simulink model "eHStest"  (R2020b)
settings: Solver=ode4  StartTime=0.0  StopTime=inf  FixedStep=Ts  RelTol=1e-3
PostLoadFcn:
  | Two_Level_Inverter_params;
InitFcn:
  | Two_Level_Inverter_params;
values from neighbouring files (symbols this model uses):
  FilterDenominator = discreteFilterc.Denominator{1}    [Two_Level_Inverter_params.m]
  FilterNumerator = discreteFilterc.Numerator{1}(2)    [Two_Level_Inverter_params.m]
  Ts = 50e-6 * 5*4    (= 0.001)    [Two_Level_Inverter_params.m]
  Udc = 650    [Two_Level_Inverter_params.m]
undefined symbols (not defined in the file or in its folder): eHSx128m_Gen4_C0D8FBCEC0D8FBCE, EX, VC707_2
libraries: powerlib_meascontrol x16, dspstat3 x8, rtlab x6, rteventslib x6, rtio_opalrt_common x5, efs_cpuhilios_crtl_lib x2, cpuhilios_lib x1, ehsCpuLib x1
settings Model: Creator=Jun Zhang  LastModifiedBy=Jun.Zhang
settings SolverCC: SolverJacobianMethodControl=FullAnalytical
settings OptimizationCC: BlockReduction=off  OptimizeBlockIOStorage=off  LocalBlockOutputs=off

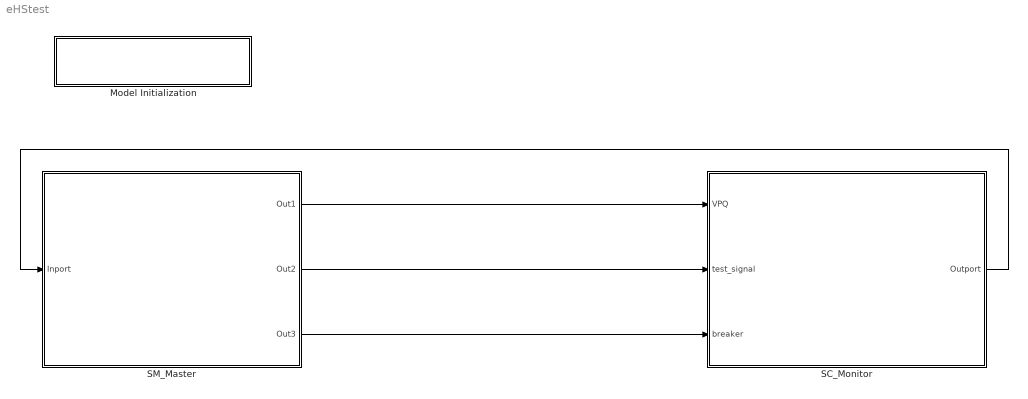
== system eHStest ==
  Model Initialization : Subsystem  AncestorBlock=artemis/Tools /Misc/Model Initialization  mask(Model Functions){InitFcnX=Two_Level_Inverter_params;, prel=off, posl=on, inif=on, strf=off}
      mask prompts: InitFcnX "Initialisation"; prel "Preload Function"; posl "PostLoad Function"; inif "InitFcn"; strf "StartFcn"
      mask init:
      | currentBlock = gcb;
      | root = bdroot(currentBlock);
      | 
      | if ~strcmp(get_param(root,'BlockDiagramType'),'library')
      |     if prel==1
      |         set_param(root, 'PreLoadFcn', InitFcnX);
      |     else
      |         set_param(root, 'PreLoadFcn', '');
      |     end
      |     if inif==1
      |         set_param(root, 'InitFcn', InitFcnX);
      |     else
      |         set_param(root, 'InitFcn', '');
      |     end
      |     if strf==1
      |         set_param(root, 'StartFcn', InitFcnX);
      |     else
      |         set_param(root, 'StartFcn', '');
      |     end
      |     if posl==1
      |         set_param(root, 'PostLoadFcn', InitFcnX);
      |     else
      |         set_param(root, 'PostLoadFcn', '');
      |     end
      | end
      | 
      | pos = get_param(currentBlock, 'Position');
      | width = pos(3) - pos(1); height = pos(4) - pos(2);
      | txt = [ upper(root) '\n' '- InitFcn. . . . . '  get_param(root, 'InitFcn') ];
      settings: CopyFcn=set_param(gcb,'LinkStatus','inactive')
      mask Display: text(5, height*0.5, txt, 'horizontalAlignment', 'left', 'verticalAlignment', 'middle') ;
  SC_Monitor : Subsystem
  SM_Master : Subsystem
  wires:
  SM_Master/1(Out1) -> SC_Monitor/1(VPQ)
  SM_Master/3(Out3) -> SC_Monitor/3(breaker)
  SM_Master/2(Out2) -> SC_Monitor/2(test_signal)
  SC_Monitor/1(Outport) -> SM_Master/1(Inport)

== system eHStest/Model Initialization ==

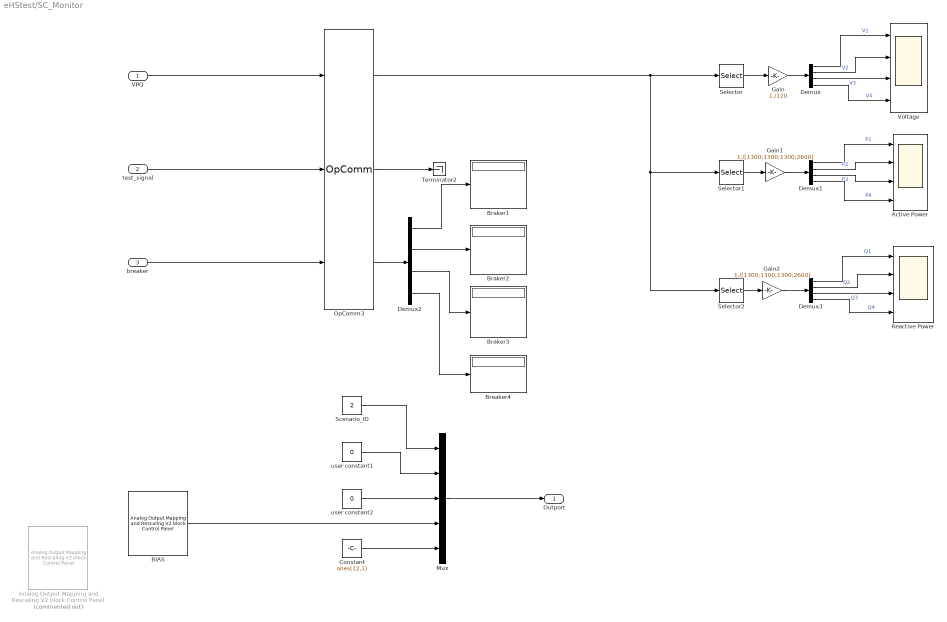
== system eHStest/SC_Monitor ==
  VPQ : Inport
  test_signal : Inport  Port=2
  breaker : Inport  Port=3
  Active Power : Scope  NumInputPorts=4
  Analog Output Mapping and Rescaling V2 block Control Panel : efs_cpuhilios_crtl_lib/Analog Output Mapping and  Rescaling V2 block Control Panel  Commented=on  controllerName='OpCtrl'  aomrVersion=V2  numberOfSourcesV1=0  numberOfSourcesV2=1  inputName0=Custom List  list0={'UserAnalogOut1', 'UserAnalogOut2', 'UserAnalogOut3', 'UserAnalogOut4'}  inputName1=Custom List  list1={'ehs1.Y1', 'ehs1.Y2', 'ehs1.Y3', 'ehs1.Y4', 'ehs1.Y5', 'ehs1.Y6', 'ehs1.Y7', 'ehs1.Y8', 'ehs1.Y9', 'ehs1.Y10', 'ehs1.Y11', 'ehs1.Y12', 'ehs1.Y13', 'ehs1.Y14', 'ehs1.Y15', 'ehs1.Y16', 'ehs1.Y17','ehs1.Y18','ehs1.Y19','ehs1.Y20','ehs1.Y21','ehs1.Y22','ehs1.Y23','ehs1.Y24','ehs1.Y25','ehs1.Y26','ehs1.Y27','ehs1.Y28','ehs1.Y29','ehs1.Y30'}  inputName2=Custom List  list2={}  inputName3=Custom List  list3={}  inputName4=Custom List  list4={}  inputName5=Custom List  list5={}  inputName6=Custom List  list6={}  inputName7=Custom List  list7={}  inputName8=Custom List  list8={}  mappingData={ 'ehs1.Y1', '16/40', '0', '-10', '10'; 'ehs1.Y2', '16/40', '0', '-10', '10'; 'ehs1.Y3', '16/40', '0', '-10', '10'; 'ehs1.Y4', '16/400', '0', '-10', '10'; 'ehs1.Y5', '16/400', '0', '-10', '10'; 'ehs1.Y6', '16/400', '0', '-10', '10'; 'Unassigned', '16/400', '0', '-10', '10'; 'Unassigned', '16/400', '0', '-10', '10'; 'ehs1.Y7', '16/40', '0', '-10', '10'; 'ehs1.Y8', '16/40', '0', '-10', '10'; 'ehs1.Y9', '16/40', '0', '-10', '10'; 'ehs1.Y10', '16/400', '0', '-10', '10'; 'ehs1.Y11', '16/400', '0', '-10', '10'; 'ehs1.Y12', '16/400', '0', '-10', '10'; 'ehs1.Y13', '16/400', '0', '-10', '10'; 'ehs1.Y14', '16/400', '0', '-10', '10'; 'ehs1.Y15', '16/40', '0', '-10', '10'; 'ehs1.Y16', '16/40', '0', '-10', '10'; 'ehs1.Y17', '16/40', '0', '-10', '10'; 'ehs1.Y18', '16/400', '0', '-10', '10'; 'ehs1.Y19', '16/400', '0', '-10', '10'; 'ehs1.Y20', '16/400', '0', '-10', '10'; 'ehs1.Y21', '16/400', '0', '-10', '10'; 'ehs1.Y22', '16/400', '0', '-10', '10'; 'ehs1.Y23', '16/40', '0', '-10', '10'; 'ehs1.Y24', '16/40', '0', '-10', '10'; 'ehs1.Y25', '16/40', '0', '-10', '10'; 'ehs1.Y26', '16/400', '0', '-10', '10'; 'ehs1.Y27', '16/400', '0', '-10', '10'; 'ehs1.Y28', '16/400', '0', '-10', '10'; 'ehs1.Y29', '16/400', '0', '-10', '10'; 'ehs1.Y30', '16/400', '0', '-10', '10' }  wholeConfig=[1024 1025 1026 1027 1028 1029 0 0 1030 1031 1032 1033 1034 1035 1036 1037 1038 1039 1040 1041 1042 1043 1044 1045 1046 1047 1048 1049 1050 1051 1052 1053 0.4 0.4 0.4 0.04 0.04 0.04 0.04 0.04 0.4 0.4 0.4 0.04 0.04 0.04 0.04 0.04 0.4 0.4 0.4 0.04 0.04 0.04 0.04 0.04 0.4 0.4 0.4 0.04 0.04 0.04 0.04 0.04 0 0 0 0 0 0 0 0 0 0 0 0 0 0 0 0 0 0 0 0 0 0 0 0 0 0 0 0 0 0 0 0 10 10 10 10 10 10 10 10 10 10 10 10 10 10 10 10 10 10 10 10 10 10 10 10 10 10 10 10 10 10 10 10 -10 -10 -10 -10 -10 -10 -10 -10 -10 -10 -10 -10 -10 -10 -10 -10 -10 -10 -10 -10 -10 -10 -10 -10 -10 -10 -10 -10 -10 -10 -10 -10]
      link override wholeConfig: Value="[ 1024  1025  1026  1027  1028  1029     0     0  1030  1031  1032  1033  1034  1035  1036  1037  1038  1039  1040  1041  1042  1043  1044  1045  1046  1047  1048  1049  1050  1051  1052  1053 16/40 16/40 16/40 16/400 16/400 16/400 16/400 16/400 16/40 16/40 16/40 16/400 16/400 16/400 16/400 16/400 16/40 16/40 16/40 16/400 16/400 16/400 16/400 16/400 16/40 16/40 16/40 16/400 16/400 16/400 16/400 16/400 0 0 0 0 0 0 0 0 0 0 0 0 0 0 0 0 0 0 0 0 0 0 0 0 0 0 0 0 0 0 0 0 10 10 10 10 10 10 10 10 10 10 10 10 10 10 10 10 10 10 10 10 10 10 10 10 10 10 10 10 10 10 10 10 -10 -10 -10 -10 -10 -10 -10 -10 -10 -10 -10 -10 -10 -10 -10 -10 -10 -10 -10 -10 -10 -10 -10 -10 -10 -10 -10 -10 -10 -10 -10 -10 ]"
  BIAS : efs_cpuhilios_crtl_lib/Analog Output Mapping and  Rescaling V2 block Control Panel  controllerName='OpCtrl'  aomrVersion=V2  numberOfSourcesV1=0  numberOfSourcesV2=1  inputName0=Custom List  list0={'UserAnalogOut1', 'UserAnalogOut2', 'UserAnalogOut3', 'UserAnalogOut4'}  inputName1=Custom List  list1={'ehs1.Y1', 'ehs1.Y2', 'ehs1.Y3', 'ehs1.Y4', 'ehs1.Y5', 'ehs1.Y6', 'ehs1.Y7', 'ehs1.Y8', 'ehs1.Y9', 'ehs1.Y10', 'ehs1.Y11', 'ehs1.Y12', 'ehs1.Y13', 'ehs1.Y14', 'ehs1.Y15', 'ehs1.Y16', 'ehs1.Y17','ehs1.Y18','ehs1.Y19','ehs1.Y20','ehs1.Y21','ehs1.Y22','ehs1.Y23','ehs1.Y24','ehs1.Y25','ehs1.Y26','ehs1.Y27','ehs1.Y28','ehs1.Y29','ehs1.Y30'}  inputName2=Custom List  list2={}  inputName3=Custom List  list3={}  inputName4=Custom List  list4={}  inputName5=Custom List  list5={}  inputName6=Custom List  list6={}  inputName7=Custom List  list7={}  inputName8=Custom List  list8={}  mappingData={ 'ehs1.Y1', '16/40', '0.003', '-10', '10'; 'ehs1.Y2', '16/40', '0.0035', '-10', '10'; 'ehs1.Y3', '16/40', '0.0115', '-10', '10'; 'ehs1.Y4', '16/400', '-0.0113', '-10', '10'; 'ehs1.Y5', '16/400', '0.0113', '-10', '10'; 'ehs1.Y6', '16/400', '0.0114', '-10', '10'; 'Unassigned', '16/400', '0.0165', '-10', '10'; 'Unassigned', '16/400', '0.0075', '-10', '10'; 'ehs1.Y7', '16/40', '0.005', '-10', '10'; 'ehs1.Y8', '16/40', '0.005', '-10', '10'; 'ehs1.Y9', '16/40', '0.005', '-10', '10'; 'ehs1.Y10', '16/400', '-0.0025', '-10', '10'; 'ehs1.Y11', '16/400', '-0.021', '-10', '10'; 'ehs1.Y12', '16/400', '-0.021', '-10', '10'; 'ehs1.Y13', '16/400', '-0.02', '-10', '10'; 'ehs1.Y14', '16/400', '-0.027', '-10', '10'; 'ehs1.Y15', '16/40', '0.003', '-10', '10'; 'ehs1.Y16', '16/40', '0.004', '-10', '10'; 'ehs1.Y17', '16/40', '0.0045', '-10', '10'; 'ehs1.Y18', '16/400', '-0.011', '-10', '10'; 'ehs1.Y19', '16/400', '-0.031', '-10', '10'; 'ehs1.Y20', '16/400', '-0.0315', '-10', '10'; 'ehs1.Y21', '16/400', '-0.034', '-10', '10'; 'ehs1.Y22', '16/400', '-0.030', '-10', '10'; 'ehs1.Y23', '16/40', '-0.0015', '-10', '10'; 'ehs1.Y24', '16/40', '0.00405', '-10', '10'; 'ehs1.Y25', '16/40', '0.002', '-10', '10'; 'ehs1.Y26', '16/400', '-0.0105', '-10', '10'; 'ehs1.Y27', '16/400', '0.022', '-10', '10'; 'ehs1.Y28', '16/400', '0.018', '-10', '10'; 'ehs1.Y29', '16/400', '0.0205', '-10', '10'; 'ehs1.Y30', '16/400', '0.0205', '-10', '10' }  wholeConfig=[1024 1025 1026 1027 1028 1029 0 0 1030 1031 1032 1033 1034 1035 1036 1037 1038 1039 1040 1041 1042 1043 1044 1045 1046 1047 1048 1049 1050 1051 1052 1053 0.4 0.4 0.4 0.04 0.04 0.04 0.04 0.04 0.4 0.4 0.4 0.04 0.04 0.04 0.04 0.04 0.4 0.4 0.4 0.04 0.04 0.04 0.04 0.04 0.4 0.4 0.4 0.04 0.04 0.04 0.04 0.04 0.003 0.0035 0.0115 -0.0113 0.0113 0.0114 0.0165 0.0075 0.005 0.005 0.005 -0.0025 -0.021 -0.021 -0.02 -0.027 0.003 0.004 0.0045 -0.011 -0.031 -0.0315 -0.034 -0.03 -0.0015 0.00405 0.002 -0.0105 0.022 0.018 0.0205 0.0205 10 10 10 10 10 10 10 10 10 10 10 10 10 10 10 10 10 10 10 10 10 10 10 10 10 10 10 10 10 10 10 10 -10 -10 -10 -10 -10 -10 -10 -10 -10 -10 -10 -10 -10 -10 -10 -10 -10 -10 -10 -10 -10 -10 -10 -10 -10 -10 -10 -10 -10 -10 -10 -10]
      link override wholeConfig: Value="[ 1024  1025  1026  1027  1028  1029     0     0  1030  1031  1032  1033  1034  1035  1036  1037  1038  1039  1040  1041  1042  1043  1044  1045  1046  1047  1048  1049  1050  1051  1052  1053 16/40 16/40 16/40 16/400 16/400 16/400 16/400 16/400 16/40 16/40 16/40 16/400 16/400 16/400 16/400 16/400 16/40 16/40 16/40 16/400 16/400 16/400 16/400 16/400 16/40 16/40 16/40 16/400 16/400 16/400 16/400 16/400 0.003 0.0035 0.0115 -0.0113 0.0113 0.0114 0.0165 0.0075 0.005 0.005 0.005 -0.0025 -0.021 -0.021 -0.02 -0.027 0.003 0.004 0.0045 -0.011 -0.031 -0.0315 -0.034 -0.030 -0.0015 0.00405 0.002 -0.0105 0.022 0.018 0.0205 0.0205 10 10 10 10 10 10 10 10 10 10 10 10 10 10 10 10 10 10 10 10 10 10 10 10 10 10 10 10 10 10 10 10 -10 -10 -10 -10 -10 -10 -10 -10 -10 -10 -10 -10 -10 -10 -10 -10 -10 -10 -10 -10 -10 -10 -10 -10 -10 -10 -10 -10 -10 -10 -10 -10 ]"
  Braker1 : Display
  Braker2 : Display
  Braker3 : Display
  Breaker4 : Display
  Constant : Constant  Value=ones(12,1)
  Demux{,1..3} (4 alike) : Demux
  Gain : Gain  Gain=1./120
  Gain1 : Gain  Gain=1./[1300;1300;1300;2600]
  Gain2 : Gain  Gain=1./[1300;1300;1300;2600]
  Mux : Mux  Inputs=5
  OpComm3 : rtlab/OpComm  nbport=3  groupe_acq=3  subsys_rate=Ts*10  st=0  Synchronization=on  Interpolation=on  Threshold=1.0  Missed_Data=off  Sim_Time=off  Samples=off  dynSigOut=off  from_console=0  warning_done=off  writeOpCommFile=off  Offset=off
      settings: SourceProductName=RT-LAB
  Reactive Power : Scope  NumInputPorts=4
  Scenario_ID : Constant  Value=2
  Selector : Selector  InputPortWidth=12  IndexOptions=Index vector (dialog)  Indices=[1:4]  OutputSizes=1
  Selector1 : Selector  InputPortWidth=12  IndexOptions=Index vector (dialog)  Indices=[5:8]  OutputSizes=1
  Selector2 : Selector  InputPortWidth=12  IndexOptions=Index vector (dialog)  Indices=[9:12]  OutputSizes=1
  Terminator2 : Terminator
  Voltage : Scope  NumInputPorts=4
  user constant1 : Constant  Value=0
  user constant2 : Constant  Value=0
  Outport : Outport
  wires:
  VPQ/1 -> OpComm3/1
  test_signal/1 -> OpComm3/2
  breaker/1 -> OpComm3/3
  Scenario_ID/1 -> Mux/1
  Mux/1 -> Outport/1
  user constant1/1 -> Mux/2
  user constant2/1 -> Mux/3
  BIAS/1 -> Mux/4
  OpComm3/3 -> Demux2/1
  OpComm3/1 -> Selector2/1, Selector1/1, Selector/1
  OpComm3/2 -> Terminator2/1
  Constant/1 -> Mux/5
  Demux2/1 -> Braker1/1
  Demux2/2 -> Braker2/1
  Demux2/3 -> Braker3/1
  Demux2/4 -> Breaker4/1
  Selector/1 -> Gain/1
  Demux/1 -> Voltage/1  "V1"
  Demux/2 -> Voltage/2  "V2"
  Demux/3 -> Voltage/3  "V3"
  Demux/4 -> Voltage/4  "V4"
  Demux1/4 -> Active Power/4  "P4"
  Demux1/3 -> Active Power/3  "P3"
  Demux1/2 -> Active Power/2  "P2"
  Selector1/1 -> Gain1/1
  Demux1/1 -> Active Power/1  "P1"
  Demux3/3 -> Reactive Power/3  "Q3"
  Selector2/1 -> Gain2/1
  Demux3/4 -> Reactive Power/4  "Q4"
  Demux3/1 -> Reactive Power/1  "Q1"
  Demux3/2 -> Reactive Power/2  "Q2"
  Gain/1 -> Demux/1
  Gain1/1 -> Demux1/1
  Gain2/1 -> Demux3/1

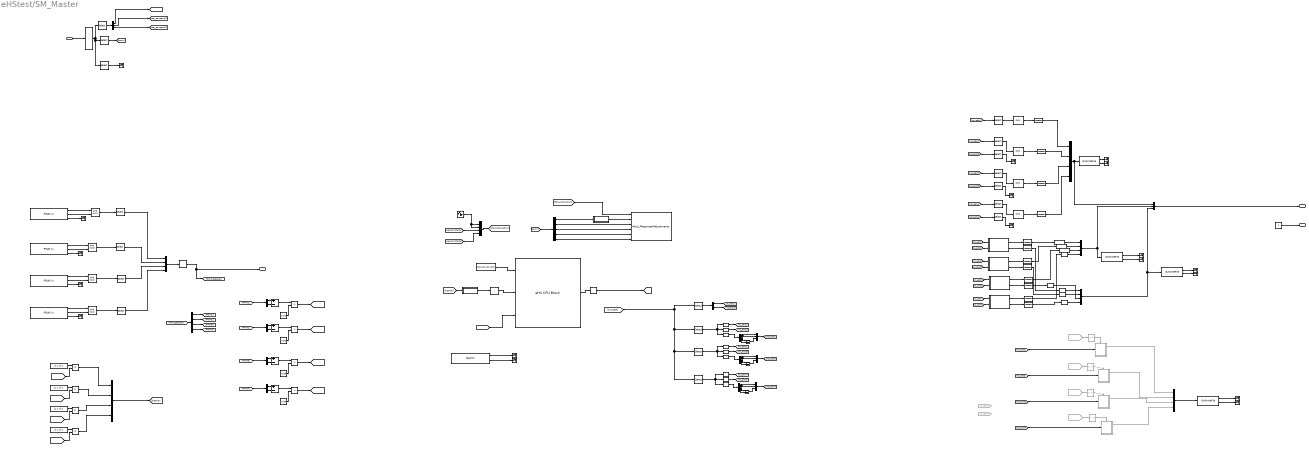
== system eHStest/SM_Master ==
  note: output
  note: model core
  note: breaker control
  note: use Vo3 and Vo4 will cause incorrect frequency measurement
  Inport : Inport
  AOMR_Trigger : Subsystem
  Add : Sum  Inputs=--
  Add1 : Sum  Inputs=--
  Add2 : Sum  Inputs=--
  Analog Output Mapping & Rescaling Controller : cpuhilios_lib/Aout_Mapping&Adjustments  ChNum=32 (2 Aout mezz)  UserAoutNum=4  block_index=1  CtrlerName='OpCtrl'  automaticPortConfiguration=off  aomrCore=AOMR Core 1  DataInId=19  LoadInId=12
      settings: AttributesFormatString=%<CtrlerName>
  Breaker control{1..4} (4 alike) : Constant  Value=[1 1 1]*1
  Breaker_Trigger : Subsystem
  Bus Creator : BusCreator  Inputs=4
  Bus Creator1 : BusCreator  Inputs=4
  Constant : Constant  Value=[Udc Udc Udc Udc]
  Constant1 : Constant
  Constant{2..5} (4 alike) : Constant  Value=0.99
  DG1 : Subsystem
  DG2 : Subsystem
  DG3 : Subsystem
  DG4 : Subsystem
  Delay{,1..3} (4 alike) : Delay  Commented=on  DelayLength=5
  Demux : Demux  Outputs=5
  Demux1 : Demux  Outputs=3
  Demux{2..4,6..10} (8 alike) : Demux  Outputs=2
  Demux5 : Demux
  Discrete Transfer Fcn{1..12} (12 alike) : DiscreteTransferFcn  Numerator=FilterNumerator  Denominator=FilterDenominator
  From31 : From  Commented=on  GotoTag=Vo_abc3
  From32 : From  Commented=on  GotoTag=Vo_abc4
  From33 : From  Commented=on  GotoTag=Breaker2_St
  From34 : From  Commented=on  GotoTag=Breaker3_St
  From35 : From  Commented=on  GotoTag=Breaker4_St
  From37 : From  Commented=on  GotoTag=Breaker1_St
  GreaterThan{,1..3} (4 alike) : RelationalOperator  Operator=>  OutDataTypeStr=boolean  RndMeth=Simplest
  Memory : Memory
  Minus{,1..3} (4 alike) : Sum  Inputs=+-
  Moving Average{,1..7} (8 alike) : dspstat3/Moving Average  Method=Sliding window  ForgettingFactorPort=off  SpecifyWindowLength=on  WindowLength=10  ForgettingFactor=0.9  SimulateUsing=Code generation
  Mux{,1..4} (5 alike) : Mux
  Mux{5..8} (4 alike) : Mux  Inputs=3
  OpComm : rtlab/OpComm  nbport=1  groupe_acq=1  subsys_rate=0  st=0  Synchronization=on  Interpolation=on  Threshold=1.0  Missed_Data=off  Sim_Time=off  Samples=off  dynSigOut=off  from_console=1  warning_done=off  writeOpCommFile=off  Offset=off
      settings: SourceProductName=RT-LAB
  OpCtrl : rtio_opalrt_common/OpCtrl  CtrlName='OpCtrl'  boardid=0  BitstreamFilename=VC707_2-EX-0001-3_5_0_817-eHSx128m_Gen4_C0D8FBCEC0D8FBCE-4F-31.bin  numconfig=-1  mode=Master  externalClock=off  decimRtsi=0  calibIO=off  SampleTime=Ts  loadinport=-1  BoardType=VC707  SecondaryPresent=off  sync_type=Audio  scope_enable=off  fsdFileName=VC707_2-EX-0001-3_5_0_817-eHSx128m_Gen4_C0D8FBCEC0D8FBCE-4F-31.fsd  mismatch_disable=off
      settings: SourceProductName=RT-LAB I/O
  OpWriteFile1 : rtlab/DataLogging/OpWriteFile  Static_File=on  varname=V_rms  Filename=V_rms.mat  rtpath='./'  nrtpath='.\'  Acq_Group=26  file_size=[100000000]  write_offline=off  Sim_Mode=off  Nb_Samples=10  Buffer_size=100000000
      settings: SourceProductName=RT-LAB  Decimation=2
  OpWriteFile3 : rtlab/DataLogging/OpWriteFile  Static_File=on  varname=P  Filename=P.mat  rtpath='./'  nrtpath='.\'  Acq_Group=27  file_size=[100000000]  write_offline=off  Sim_Mode=off  Nb_Samples=10  Buffer_size=100000000
      settings: SourceProductName=RT-LAB  Decimation=2
  OpWriteFile4 : rtlab/DataLogging/OpWriteFile  Static_File=on  varname=Q  Filename=Q.mat  rtpath='./'  nrtpath='.\'  Acq_Group=28  file_size=[100000000]  write_offline=off  Sim_Mode=off  Nb_Samples=10  Buffer_size=100000000
      settings: SourceProductName=RT-LAB  Decimation=2
  OpWriteFile5 : rtlab/DataLogging/OpWriteFile  Static_File=on  varname=fre  Filename=fre.mat  rtpath='./'  nrtpath='.\'  Acq_Group=29  file_size=[100000000]  write_offline=off  Sim_Mode=off  Nb_Samples=10  Buffer_size=100000000
      settings: SourceProductName=RT-LAB  Decimation=2
  PWM In : rtio_opalrt_common/PWM In  CtrlName='OpCtrl'  portNb=3  FcnNos=Slot 2 Module A Subsection 1  maxCount=8  Count=8  sampleTime=0  numchan=8
      settings: AttributesFormatString=%<CtrlName>  SourceProductName=RT-LAB I/O
  PWM In1 : rtio_opalrt_common/PWM In  CtrlName='OpCtrl'  portNb=4  FcnNos=Slot 2 Module A Subsection 2  maxCount=8  Count=8  sampleTime=0  numchan=8
      settings: AttributesFormatString=%<CtrlName>  SourceProductName=RT-LAB I/O
  PWM In2 : rtio_opalrt_common/PWM In  CtrlName='OpCtrl'  portNb=5  FcnNos=Slot 2 Module A Subsection 3  maxCount=8  Count=8  sampleTime=0  numchan=8
      settings: AttributesFormatString=%<CtrlName>  SourceProductName=RT-LAB I/O
  PWM In3 : rtio_opalrt_common/PWM In  CtrlName='OpCtrl'  portNb=6  FcnNos=Slot 2 Module A Subsection 4  maxCount=8  Count=8  sampleTime=0  numchan=8
      settings: AttributesFormatString=%<CtrlName>  SourceProductName=RT-LAB I/O
  Product{,1..3} (4 alike) : Product
  RMS{1..4} (4 alike) : powerlib_meascontrol/Measurements/RMS  TrueRMS=on  Freq=60  RMSInit=120  Ts=0
  RTE Conversion : rteventslib/Signal Attributes/RTE Conversion  inputdatatype=RTE Boolean  outputdatatype=Double  compensation=Enabled  nbMaxEvents=10  sampleTime=Ts
  RTE Conversion1 : rteventslib/Signal Attributes/RTE Conversion  inputdatatype=Double  outputdatatype=RTE Boolean  compensation=Enabled  nbMaxEvents=21  sampleTime=Ts
  RTE PWM{,1..3} (4 alike) : rteventslib/Sources/RTE PWM  ShiftedTransition=Enabled  MaxEvents=10  SampleTime=Ts
  Selector{,6,8..9,21..23} (7 alike) : Selector  InputPortWidth=3  IndexOptions=Index vector (dialog)  Indices=[1]  OutputSizes=1
  Selector1 : Selector  IndexOptions=Index vector (dialog)  Indices=[164:175]  OutputSizes=1
  Selector10 : Selector  InputPortWidth=30  IndexOptions=Index vector (dialog)  Indices=[23:30]  OutputSizes=1
  Selector{11..13,19} (4 alike) : Selector  IndexOptions=Index vector (dialog)  Indices=[1:3]  OutputSizes=1
  Selector14 : Selector  IndexOptions=Index vector (dialog)  Indices=[4:6]  OutputSizes=1
  Selector15 : Selector  IndexOptions=Index vector (dialog)  Indices=[4:6]  OutputSizes=1
  Selector16 : Selector  IndexOptions=Index vector (dialog)  Indices=[4:6]  OutputSizes=1
  Selector{2..5,7,17..18} (7 alike) : Selector  IndexOptions=Index vector (dialog)  Indices=[7:8]  OutputSizes=1
  Selector20 : Selector  IndexOptions=Index vector (dialog)  Indices=[4:163]  OutputSizes=1
  Selector24 : Selector  InputPortWidth=30  IndexOptions=Index vector (dialog)  Indices=[1:6]  OutputSizes=1
  Selector25 : Selector  InputPortWidth=30  IndexOptions=Index vector (dialog)  Indices=[7:14]  OutputSizes=1
  Selector26 : Selector  InputPortWidth=30  IndexOptions=Index vector (dialog)  Indices=[15:22]  OutputSizes=1
  Sine Wave : Sin  Bias=1  Frequency=60*2*pi  SampleTime=0
  Subsystem : Subsystem  Commented=on
  Subsystem1 : Subsystem  Commented=on
  Subsystem2 : Subsystem  Commented=on
  Subsystem3 : Subsystem  Commented=on
  Terminator{,1..8,10..15,18..20} (18 alike) : Terminator
  eHS CPU Block : ehsCpuLib/eHS CPU Block  solverPerformanceFormFactor=x128  solverGeneration=Gen 4  lastSuccessfullGeneration=11-Feb-2025 10:56:58 - Circuit: Circuit_4DG_LC.slx - 4U 33SW 30Y  circuitSource=Use File on Disk  eDBSIMlist=<empty>  eDBSIMid=0  circuitFileName=Circuit_4DG_LC.slx  useExplicitTs=off  Ts_eHS=5E-7  useExplicitGs=off  Gs=0.4  validCircuitSelected=off  validSolverSelected=on  validConfigurationSet=off  validScenariosSelected=on  programmingFileGenerated=on  programmingFileName=C:/Users/Jun.Zhang/OPAL-RT/RT-LABv2023.1_Workspace/4DG_OPT_LC/models/eHStest\EFPGASIMConfig\ehsConfigEhsGen4x128SID61.mat  nbActualCpuInputs=4  actualUseRte=on  nbActualCpuGates=12  nbActualCpuOutputs=30  nbInputs=4  nbSwitches=33  nbOutputs=30  inputConfiguration=[0 0;0 1;0 2;0 3]  gateConfiguration=[2 0 0 0;2 1 0 0;2 2 0 0;2 3 0 0;2 4 0 0;2 5 0 0;2 8 0 0;2 9 0 0;2 10 0 0;2 11 0 0;2 12 0 0;2 13 0 0;0 3 0 0;0 4 0 0;0 5 0 0;2 16 0 0;2 17 0 0;2 18 0 0;2 19 0 0;2 20 0 0;2 21 0 0;0 6 0 0;0 7 0 0;0 8 0 0;2 24 0 0;2 25 0 0;2 26 0 0;2 27 0 0;2 28 0 0;2 29 0 0;0 9 0 0;0 10 0 0;0 11 0 0]  actualTs=4.9e-07  minTs=4.9e-07  enableResetPin=off  nbSWG=0  inputAutoMode='on'  useSWG=off  useRtEvents=on  nbEvents=10  useScenarioFeature=on  xlsFileName=C:\Users\Jun.Zhang\OPAL-RT\RT-LABv2023.1_Workspace\4DG_OPT_LC\models\eHStest\Circuit_4DG_LC.slx.xlsx  xlsSheetNumber=1  nbUsedScenarios=4  nbMaxScenarios=11  enableThermalLoss=off  thermalLossAutoMode=on  thermalLossNbArmsEnabled=0  ConductionTableSwitch1=0  ConductionTable2Switch1=0  ConductionSwitchBPCur1=0  ConductionSwitchBPTemp1=0  TurnOnTableSwitch1=0  TurnOffTableSwitch1=0  TurnOnOffSwitchBPCur1=0  TurnOnOffSwitchBPVolt1=0  TurnOnOffSwitchBPTemp1=0  ConductionTableDiode1=0  ConductionTable2Diode1=0  ConductionDiodeBPCur1=0  ConductionDiodeBPTemp1=0  TurnOnTableDiode1=0  TurnOffTableDiode1=0  TurnOnOffDiodeBPCur1=0  TurnOnOffDiodeBPVolt1=0  TurnOnOffDiodeBPTemp1=0  ConductionTableSwitch2=0  ConductionTable2Switch2=0  ConductionSwitchBPCur2=0  ConductionSwitchBPTemp2=0  TurnOnTableSwitch2=0  TurnOffTableSwitch2=0  TurnOnOffSwitchBPCur2=0  TurnOnOffSwitchBPVolt2=0  TurnOnOffSwitchBPTemp2=0  ConductionTableDiode2=0  ConductionTable2Diode2=0  ConductionDiodeBPCur2=0  ConductionDiodeBPTemp2=0  TurnOnTableDiode2=0  TurnOffTableDiode2=0  TurnOnOffDiodeBPCur2=0  TurnOnOffDiodeBPVolt2=0  TurnOnOffDiodeBPTemp2=0  ConductionTableSwitch3=0  ConductionTable2Switch3=0  ConductionSwitchBPCur3=0  ConductionSwitchBPTemp3=0  TurnOnTableSwitch3=0  TurnOffTableSwitch3=0  TurnOnOffSwitchBPCur3=0  TurnOnOffSwitchBPVolt3=0  TurnOnOffSwitchBPTemp3=0  ConductionTableDiode3=0  ConductionTable2Diode3=0  ConductionDiodeBPCur3=0  ConductionDiodeBPTemp3=0  TurnOnTableDiode3=0  TurnOffTableDiode3=0  TurnOnOffDiodeBPCur3=0  TurnOnOffDiodeBPVolt3=0  TurnOnOffDiodeBPTemp3=0  ConductionTableSwitch4=0  ConductionTable2Switch4=0  ConductionSwitchBPCur4=0  ConductionSwitchBPTemp4=0  TurnOnTableSwitch4=0  TurnOffTableSwitch4=0  TurnOnOffSwitchBPCur4=0  TurnOnOffSwitchBPVolt4=0  TurnOnOffSwitchBPTemp4=0  ConductionTableDiode4=0  ConductionTable2Diode4=0  ConductionDiodeBPCur4=0  ConductionDiodeBPTemp4=0  TurnOnTableDiode4=0  TurnOffTableDiode4=0  TurnOnOffDiodeBPCur4=0  TurnOnOffDiodeBPVolt4=0  TurnOnOffDiodeBPTemp4=0  useExplicitCommPort=off  ctrlName='OpCtrl'  automaticPortConfiguration=on  ehsCore=Ehs Core 1  solverFormFactor=x128  commPortNumbers=[1 2 1 2:1:2+8 1]  cpuInputsPortNumber=1  cpuGatesPortNumber=[2 3 4 5 6 7 8 9 10 34 35 36 37 38 39 40 41 42]  cpuOutputsPortNumber=1  ehsConfigPortNumber=1  rstAndScenarioPortNumber=2  swgDatainPort=27  thermalLossDataInPort=28  thermalLossDataOutPort=19  thermalLossLoadInPort=25  enCustomFirmwareConfiguration=off  firmwareCustomInputSourcesConfig=0  firmwareDefaultInputSourcesConfig={'CPU Model',0,128;'Analog Input',1,32;'Sine Wave Generator',3,32;'Saturable Transformer',2,32}  firmwareCustomGateSourcesConfig=0  firmwareDefaultGateSourcesConfig={'CPU Model',0,72;'Digital Input',2,64;'PWM',1,32}
      link override ehsCpuOutputs: sampleTime=Ts
      settings: AttributesFormatString=%<CtrlName>
  Out1 : Outport
  Out2 : Outport  Port=2
  Out3 : Outport  Port=3
  wires:
  Constant/1 -> eHS CPU Block/1
  OpCtrl/1 -> Terminator/1
  OpCtrl/2 -> Terminator1/1
  Memory/1 -> [bus_data]  "bus_data"
  Inport/1 -> OpComm/1
  OpComm/1 -> Selector1/1, Selector20/1, Selector19/1
  Demux1/1 -> [Scenario_ID]
  Demux1/2 -> [user_constant1]
  Demux1/3 -> [user_constant2]
  eHS CPU Block/1 -> Memory/1
  [CPU_Modulation] -> Analog Output Mapping & Rescaling Controller/1
  [aomr] -> Demux/1
  Demux/1 -> AOMR_Trigger/1(In1)
  Demux/2 -> Analog Output Mapping & Rescaling Controller/3
  Demux/3 -> Analog Output Mapping & Rescaling Controller/4
  Demux/4 -> Analog Output Mapping & Rescaling Controller/5
  Demux/5 -> Analog Output Mapping & Rescaling Controller/6
  Selector20/1 -> [aomr]
  Selector19/1 -> Demux1/1
  AOMR_Trigger/1(Out1) -> Analog Output Mapping & Rescaling Controller/2
  [Scenario_ID] -> eHS CPU Block/3
  Selector1/1 -> Terminator11/1
  RTE Conversion1/1 -> eHS CPU Block/2
  Sine Wave/1 -> Mux2/2, Mux2/1
  Mux2/1 -> [CPU_Modulation]
  [breaker] -> Breaker_Trigger/1(In1)
  Breaker_Trigger/1(Out1) -> RTE Conversion1/1
  [user_constant2] -> Mux2/4
  [user_constant1] -> Mux2/3
  Constant1/1 -> Out2/1
  RTE Conversion/1 -> Out3/1, [PWM_Breaker]
  Mux1/1 -> [breaker]
  OpWriteFile3/1 -> Terminator3/1
  [Vpcc_abc2] -> Selector9/1
  [Vo_abc4] -> DG4/1(Vabc)
  DG1/1(P) -> Discrete Transfer Fcn2/1  "Pdg1"
  Selector7/1 -> Demux9/1
  Selector24/1 -> Demux8/1
  Add/1 -> Mux5/3
  Discrete Transfer Fcn7/1 -> Bus Creator/3
  [Io_abc4] -> DG4/2(iabc)
  Selector9/1 -> Terminator18/1
  RMS1/1 -> Discrete Transfer Fcn6/1
  OpWriteFile4/2 -> Terminator12/1
  [Vo_abc2] -> Selector6/1
  Demux3/1 -> Mux5/1, Add/1
  Discrete Transfer Fcn4/1 -> Moving Average2/1
  Selector10/1 -> Selector7/1, Selector13/1, Selector16/1
  [Vo_abc4] -> Selector22/1
  Bus Creator/1 -> Mux8/1, OpWriteFile1/1  "V_rms"
  Discrete Transfer Fcn8/1 -> Bus Creator/4
  Selector14/1 -> [Vo_abc2]
  Mux3/1 -> Mux8/2, OpWriteFile3/1  "P"
  [Io_abc3] -> DG3/2(iabc)
  DG4/1(P) -> Discrete Transfer Fcn11/1  "Pdg2"
  Discrete Transfer Fcn10/1 -> Moving Average5/1
  Selector21/1 -> Terminator19/1
  [Vo_abc1] -> Selector/1
  Selector8/1 -> RMS3/1
  RMS3/1 -> Discrete Transfer Fcn7/1
  OpWriteFile3/2 -> Terminator2/1
  Demux9/2 -> Add2/2, Mux7/2
  Selector6/1 -> RMS2/1
  DG3/1(P) -> Discrete Transfer Fcn9/1  "Pdg3"
  Discrete Transfer Fcn5/1 -> Moving Average7/1
  Mux5/1 -> [Vpcc_abc3]
  Selector/1 -> RMS1/1
  OpWriteFile1/2 -> Terminator10/1
  DG2/1(P) -> Discrete Transfer Fcn4/1  "Pdg2"
  Demux9/1 -> Mux7/1, Add2/1
  Discrete Transfer Fcn11/1 -> Moving Average4/1
  Selector22/1 -> RMS4/1
  DG2/2(Q) -> Discrete Transfer Fcn5/1  "Qdg2"
  [Io_abc1] -> DG1/2(iabc)
  OpWriteFile4/1 -> Terminator13/1
  DG3/2(Q) -> Discrete Transfer Fcn10/1  "Qdg1"
  Selector13/1 -> [Io_abc4]
  Mux7/1 -> [Vpcc_abc4]
  Discrete Transfer Fcn9/1 -> Moving Average3/1
  Selector11/1 -> [Io_abc2]
  Selector16/1 -> [Vo_abc4]
  [bus_data] -> Selector10/1, Selector26/1, Selector25/1, Selector24/1
  Selector26/1 -> Selector18/1, Selector12/1, Selector15/1
  [Vpcc_abc3] -> Selector21/1
  Discrete Transfer Fcn6/1 -> Bus Creator/1
  Discrete Transfer Fcn3/1 -> Moving Average6/1
  Selector12/1 -> [Io_abc3]
  [Vo_abc1] -> DG1/1(Vabc)
  Selector25/1 -> Selector11/1, Selector14/1, Selector17/1
  RMS4/1 -> Discrete Transfer Fcn8/1
  [Io_abc2] -> DG2/2(iabc)
  Discrete Transfer Fcn2/1 -> Moving Average/1
  OpWriteFile1/1 -> Terminator6/1
  DG1/2(Q) -> Discrete Transfer Fcn3/1  "Qdg1"
  Demux3/2 -> Add/2, Mux5/2
  Selector15/1 -> [Vo_abc3]
  OpWriteFile5/2 -> Terminator14/1
  [Vo_abc3] -> DG3/1(Vabc)
  Bus Creator1/1 -> OpWriteFile5/1  "fre"
  Demux4/2 -> Add1/2, Mux6/2
  [Vo_abc2] -> DG2/1(Vabc)
  Demux8/1 -> [Io_abc1]
  [Vo_abc3] -> Selector8/1
  Selector23/1 -> Terminator20/1
  DG4/2(Q) -> Discrete Transfer Fcn12/1  "Qdg2"
  Mux4/1 -> Mux8/3, OpWriteFile4/1  "Q"
  Selector18/1 -> Demux3/1
  Discrete Transfer Fcn12/1 -> Moving Average1/1
  Discrete Transfer Fcn1/1 -> Bus Creator/2
  Selector17/1 -> Demux4/1
  Add1/1 -> Mux6/3
  Mux6/1 -> [Vpcc_abc2]
  Demux8/2 -> [Vo_abc1]
  OpWriteFile5/1 -> Terminator15/1
  [Vpcc_abc4] -> Selector23/1
  Add2/1 -> Mux7/3
  Demux4/1 -> Mux6/1, Add1/1
  RMS2/1 -> Discrete Transfer Fcn1/1
  PWM In3/1 -> RTE PWM3/1
  Constant4/1 -> GreaterThan2/2
  PWM In2/2 -> RTE PWM2/2
  [Breaker3_St] -> Product1/2
  PWM In1/3 -> Terminator5/1
  [PWM4] -> Demux7/1
  Demux5/4 -> [PWM4]
  Constant3/1 -> GreaterThan1/2
  Demux5/1 -> [PWM1]
  [PWM3] -> Demux6/1
  PWM In2/1 -> RTE PWM2/1
  Demux2/2 -> Minus/2
  Constant2/1 -> GreaterThan/2
  Product/1 -> Mux1/2
  Selector3/1 -> Mux/3
  PWM In1/2 -> RTE PWM1/2
  Minus1/1 -> GreaterThan1/1
  Demux7/1 -> Minus2/1
  Demux6/1 -> Minus1/1
  RTE PWM3/1 -> Selector4/1
  PWM In/1 -> RTE PWM/1
  GreaterThan2/1 -> [Breaker4_St]
  Minus2/1 -> GreaterThan2/1
  Selector5/1 -> Mux/1
  PWM In3/3 -> Terminator8/1
  [PWM_Breaker] -> Demux5/1
  [Breaker2_St] -> Product/2
  PWM In/2 -> RTE PWM/2
  Breaker control2/1 -> Product/1
  Breaker control4/1 -> Product2/1
  PWM In2/3 -> Terminator7/1
  Product1/1 -> Mux1/3
  PWM In1/1 -> RTE PWM1/1
  RTE PWM1/1 -> Selector2/1
  Demux5/2 -> [PWM2]
  Product2/1 -> Mux1/4
  PWM In/3 -> Terminator4/1
  Breaker control3/1 -> Product1/1
  Minus/1 -> GreaterThan/1
  Demux5/3 -> [PWM3]
  [PWM2] -> Demux2/1
  Demux2/1 -> Minus/1
  Demux6/2 -> Minus1/2
  Mux/1 -> RTE Conversion/1
  GreaterThan/1 -> [Breaker2_St]
  Selector4/1 -> Mux/4
  GreaterThan1/1 -> [Breaker3_St]
  Selector2/1 -> Mux/2
  Demux7/2 -> Minus2/2
  RTE PWM2/1 -> Selector3/1
  RTE PWM/1 -> Selector5/1
  [Breaker4_St] -> Product2/2
  PWM In3/2 -> RTE PWM3/2
  Moving Average/1 -> Mux3/1
  Moving Average2/1 -> Mux3/2
  Moving Average3/1 -> Mux3/3
  Moving Average4/1 -> Mux3/4
  Moving Average1/1 -> Mux4/4
  Moving Average5/1 -> Mux4/3
  Moving Average6/1 -> Mux4/1
  Moving Average7/1 -> Mux4/2
  [Vo_abc2] -> Subsystem/1(abc)
  Subsystem/1(Freq) -> Bus Creator1/2
  From33/1 -> Delay1/1
  [Vo_abc1] -> Subsystem1/1(abc)
  Subsystem1/1(Freq) -> Bus Creator1/1
  GreaterThan3/1 -> [Breaker1_St]
  Constant5/1 -> GreaterThan3/2
  Demux10/1 -> Minus3/1
  Demux10/2 -> Minus3/2
  Minus3/1 -> GreaterThan3/1
  [PWM1] -> Demux10/1
  From37/1 -> Delay/1
  Delay/1 -> Subsystem1/Enable
  Delay1/1 -> Subsystem/Enable
  [Vpcc_abc3] -> Subsystem2/1(abc)
  Subsystem2/1(Freq) -> Bus Creator1/3
  From34/1 -> Delay2/1
  Delay2/1 -> Subsystem2/Enable
  [Vpcc_abc4] -> Subsystem3/1(abc)
  Subsystem3/1(Freq) -> Bus Creator1/4
  From35/1 -> Delay3/1
  Delay3/1 -> Subsystem3/Enable
  Mux8/1 -> Out1/1
  Breaker control1/1 -> Product3/1
  [Breaker1_St] -> Product3/2
  Product3/1 -> Mux1/1

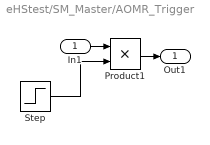
== system eHStest/SM_Master/AOMR_Trigger ==
  In1 : Inport
  Product1 : Product
  Step : Step  Time=0.5  SampleTime=0
  Out1 : Outport
  wires:
  Step/1 -> Product1/2
  In1/1 -> Product1/1
  Product1/1 -> Out1/1

== system eHStest/SM_Master/Breaker_Trigger ==
  In1 : Inport
  Product1 : Product
  Step : Step  Time=0.5  SampleTime=0
  Out1 : Outport
  wires:
  Step/1 -> Product1/2
  In1/1 -> Product1/1
  Product1/1 -> Out1/1

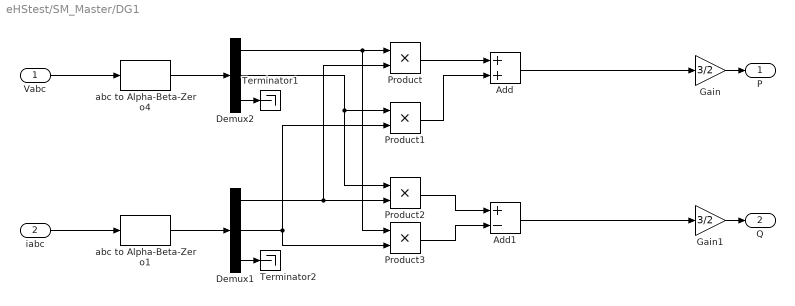
== system eHStest/SM_Master/DG1 ==
  Vabc : Inport
  iabc : Inport  Port=2
  Add : Sum
  Add1 : Sum  Inputs=+-
  Demux1 : Demux  Outputs=3
  Demux2 : Demux  Outputs=3
  Gain : Gain  Gain=3/2
  Gain1 : Gain  Gain=3/2
  Product{,1..3} (4 alike) : Product
  Terminator1 : Terminator
  Terminator2 : Terminator
  abc to Alpha-Beta-Zero1 : powerlib_meascontrol/Transformations/abc to Alpha-Beta-Zero
  abc to Alpha-Beta-Zero4 : powerlib_meascontrol/Transformations/abc to Alpha-Beta-Zero
  P : Outport  VectorParamsAs1DForOutWhenUnconnected=off
  Q : Outport  Port=2  VectorParamsAs1DForOutWhenUnconnected=off
  wires:
  iabc/1 -> abc to Alpha-Beta-Zero1/1
  Demux1/3 -> Terminator2/1
  Demux2/3 -> Terminator1/1
  Demux2/1 -> Product3/1, Product/1
  Demux1/1 -> Product/2, Product2/2
  Demux1/2 -> Product1/2, Product3/2
  Product/1 -> Add/1
  Product1/1 -> Add/2
  Demux2/2 -> Product2/1, Product1/1
  Product2/1 -> Add1/1
  Product3/1 -> Add1/2
  Vabc/1 -> abc to Alpha-Beta-Zero4/1
  abc to Alpha-Beta-Zero4/1 -> Demux2/1
  abc to Alpha-Beta-Zero1/1 -> Demux1/1
  Gain/1 -> P/1
  Gain1/1 -> Q/1
  Add/1 -> Gain/1
  Add1/1 -> Gain1/1

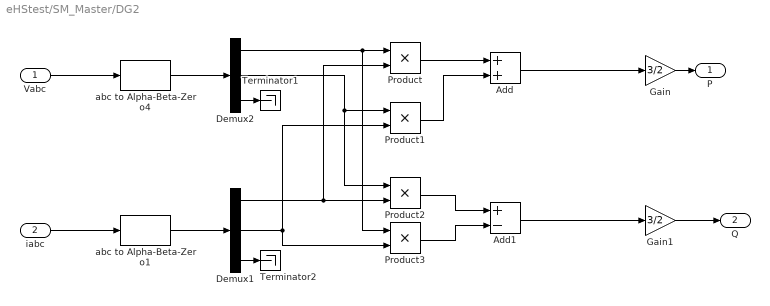
== system eHStest/SM_Master/DG2 ==
  Vabc : Inport
  iabc : Inport  Port=2
  Add : Sum
  Add1 : Sum  Inputs=+-
  Demux1 : Demux  Outputs=3
  Demux2 : Demux  Outputs=3
  Gain : Gain  Gain=3/2
  Gain1 : Gain  Gain=3/2
  Product{,1..3} (4 alike) : Product
  Terminator1 : Terminator
  Terminator2 : Terminator
  abc to Alpha-Beta-Zero1 : powerlib_meascontrol/Transformations/abc to Alpha-Beta-Zero
  abc to Alpha-Beta-Zero4 : powerlib_meascontrol/Transformations/abc to Alpha-Beta-Zero
  P : Outport  VectorParamsAs1DForOutWhenUnconnected=off
  Q : Outport  Port=2  VectorParamsAs1DForOutWhenUnconnected=off
  wires:
  iabc/1 -> abc to Alpha-Beta-Zero1/1
  Demux1/3 -> Terminator2/1
  Demux2/3 -> Terminator1/1
  Demux2/1 -> Product3/1, Product/1
  Demux1/1 -> Product/2, Product2/2
  Demux1/2 -> Product1/2, Product3/2
  Product/1 -> Add/1
  Product1/1 -> Add/2
  Demux2/2 -> Product2/1, Product1/1
  Product2/1 -> Add1/1
  Product3/1 -> Add1/2
  Add1/1 -> Gain1/1
  Vabc/1 -> abc to Alpha-Beta-Zero4/1
  abc to Alpha-Beta-Zero4/1 -> Demux2/1
  abc to Alpha-Beta-Zero1/1 -> Demux1/1
  Add/1 -> Gain/1
  Gain/1 -> P/1
  Gain1/1 -> Q/1

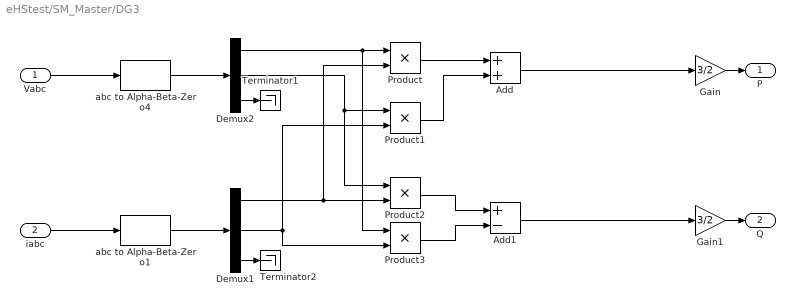
== system eHStest/SM_Master/DG3 ==
  Vabc : Inport
  iabc : Inport  Port=2
  Add : Sum
  Add1 : Sum  Inputs=+-
  Demux1 : Demux  Outputs=3
  Demux2 : Demux  Outputs=3
  Gain : Gain  Gain=3/2
  Gain1 : Gain  Gain=3/2
  Product{,1..3} (4 alike) : Product
  Terminator1 : Terminator
  Terminator2 : Terminator
  abc to Alpha-Beta-Zero1 : powerlib_meascontrol/Transformations/abc to Alpha-Beta-Zero
  abc to Alpha-Beta-Zero4 : powerlib_meascontrol/Transformations/abc to Alpha-Beta-Zero
  P : Outport  VectorParamsAs1DForOutWhenUnconnected=off
  Q : Outport  Port=2  VectorParamsAs1DForOutWhenUnconnected=off
  wires:
  iabc/1 -> abc to Alpha-Beta-Zero1/1
  Demux1/3 -> Terminator2/1
  Demux2/3 -> Terminator1/1
  Demux2/1 -> Product3/1, Product/1
  Demux1/1 -> Product/2, Product2/2
  Demux1/2 -> Product1/2, Product3/2
  Product/1 -> Add/1
  Product1/1 -> Add/2
  Demux2/2 -> Product2/1, Product1/1
  Product2/1 -> Add1/1
  Product3/1 -> Add1/2
  Vabc/1 -> abc to Alpha-Beta-Zero4/1
  abc to Alpha-Beta-Zero4/1 -> Demux2/1
  abc to Alpha-Beta-Zero1/1 -> Demux1/1
  Gain/1 -> P/1
  Gain1/1 -> Q/1
  Add/1 -> Gain/1
  Add1/1 -> Gain1/1

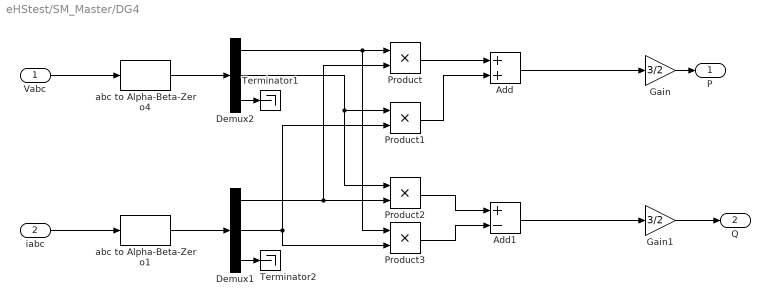
== system eHStest/SM_Master/DG4 ==
  Vabc : Inport
  iabc : Inport  Port=2
  Add : Sum
  Add1 : Sum  Inputs=+-
  Demux1 : Demux  Outputs=3
  Demux2 : Demux  Outputs=3
  Gain : Gain  Gain=3/2
  Gain1 : Gain  Gain=3/2
  Product{,1..3} (4 alike) : Product
  Terminator1 : Terminator
  Terminator2 : Terminator
  abc to Alpha-Beta-Zero1 : powerlib_meascontrol/Transformations/abc to Alpha-Beta-Zero
  abc to Alpha-Beta-Zero4 : powerlib_meascontrol/Transformations/abc to Alpha-Beta-Zero
  P : Outport  VectorParamsAs1DForOutWhenUnconnected=off
  Q : Outport  Port=2  VectorParamsAs1DForOutWhenUnconnected=off
  wires:
  iabc/1 -> abc to Alpha-Beta-Zero1/1
  Demux1/3 -> Terminator2/1
  Demux2/3 -> Terminator1/1
  Demux2/1 -> Product3/1, Product/1
  Demux1/1 -> Product/2, Product2/2
  Demux1/2 -> Product1/2, Product3/2
  Product/1 -> Add/1
  Product1/1 -> Add/2
  Demux2/2 -> Product2/1, Product1/1
  Product2/1 -> Add1/1
  Product3/1 -> Add1/2
  Add1/1 -> Gain1/1
  Vabc/1 -> abc to Alpha-Beta-Zero4/1
  abc to Alpha-Beta-Zero4/1 -> Demux2/1
  abc to Alpha-Beta-Zero1/1 -> Demux1/1
  Add/1 -> Gain/1
  Gain/1 -> P/1
  Gain1/1 -> Q/1

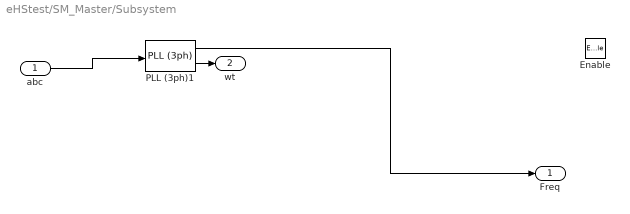
== system eHStest/SM_Master/Subsystem ==
  abc : Inport
  Enable : EnablePort
  PLL (3ph)1 : powerlib_meascontrol/PLL/PLL (3ph)  Fmin=58  Par_Init=[0, 60]  ParK=[180, 3200, 1]  TcD=Ts  MaxRateChangeFreq=12  FilterCutOffFreq=25  Ts=Ts  AGC=on
  Freq : Outport
  wt : Outport  Port=2
  wires:
  PLL (3ph)1/2 -> wt/1
  abc/1 -> PLL (3ph)1/1
  PLL (3ph)1/1 -> Freq/1

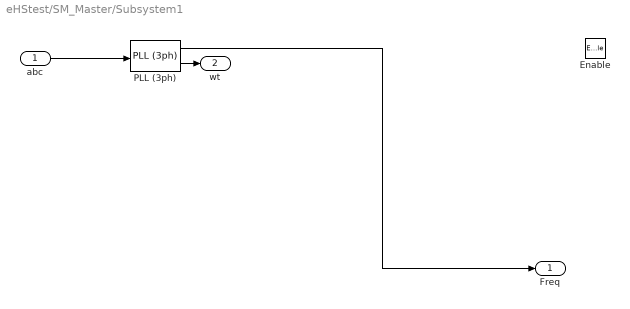
== system eHStest/SM_Master/Subsystem1 ==
  abc : Inport
  Enable : EnablePort
  PLL (3ph) : powerlib_meascontrol/PLL/PLL (3ph)  Fmin=58  Par_Init=[0, 60]  ParK=[180, 3200, 1]  TcD=Ts  MaxRateChangeFreq=12  FilterCutOffFreq=25  Ts=Ts  AGC=on
  Freq : Outport
  wt : Outport  Port=2
  wires:
  PLL (3ph)/2 -> wt/1
  PLL (3ph)/1 -> Freq/1
  abc/1 -> PLL (3ph)/1

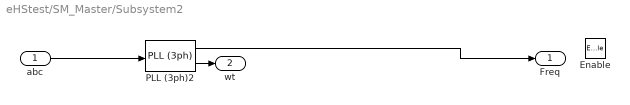
== system eHStest/SM_Master/Subsystem2 ==
  abc : Inport
  Enable : EnablePort
  PLL (3ph)2 : powerlib_meascontrol/PLL/PLL (3ph)  Fmin=58  Par_Init=[0, 60]  ParK=[180, 3200, 1]  TcD=Ts  MaxRateChangeFreq=12  FilterCutOffFreq=25  Ts=Ts  AGC=on
  Freq : Outport
  wt : Outport  Port=2
  wires:
  PLL (3ph)2/2 -> wt/1
  abc/1 -> PLL (3ph)2/1
  PLL (3ph)2/1 -> Freq/1

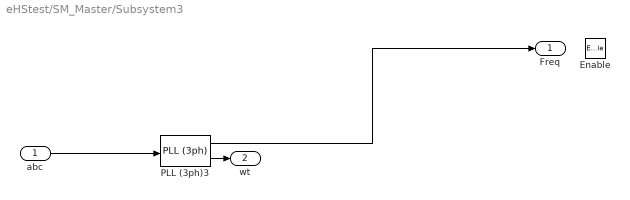
== system eHStest/SM_Master/Subsystem3 ==
  abc : Inport
  Enable : EnablePort
  PLL (3ph)3 : powerlib_meascontrol/PLL/PLL (3ph)  Fmin=58  Par_Init=[0, 60]  ParK=[180, 3200, 1]  TcD=Ts  MaxRateChangeFreq=12  FilterCutOffFreq=25  Ts=Ts  AGC=on
  Freq : Outport
  wt : Outport  Port=2
  wires:
  abc/1 -> PLL (3ph)3/1
  PLL (3ph)3/1 -> Freq/1
  PLL (3ph)3/2 -> wt/1
